simulink model "EENGquadcopter_control"  (R2018b)
settings: Solver=VariableStepAuto  StartTime=0.0  StopTime=10.0  RelTol=1e-3
values from neighbouring files (symbols this model uses):
  armLength = 0.1    [EENGquadcopter.m]
  dragFactor = 0.1    [EENGquadcopter.m]
  iX = 0.03    [EENGquadcopter.m]
  iY = 0.03    [EENGquadcopter.m]
  iZ = 0.03    [EENGquadcopter.m]
  mass = 0.25    [EENGquadcopter.m]
  om1 = 2.8    [EENGquadcopter.m]
  om2 = 3.2    [EENGquadcopter.m]
  om3 = 3.2    [EENGquadcopter.m]
  om4 = 2.8    [EENGquadcopter.m]
  phi0 = 0.0    (= 0)    [EENGquadcopter.m]    (also in EKFquadcopter-1.m = x_k0(4) + (e*(-1^count)); UKFquadcopter-1.m = xI_p(4,i))
  phiDot0 = 0.0    (= 0)    [EENGquadcopter.m]    (also in EKFquadcopter-1.m = x_k0(10) + (e*(-1^(count+1))); UKFquadcopter-1.m = xI_p(10,i))
  psi0 = 0.0    (= 0)    [EENGquadcopter.m]    (also in EKFquadcopter-1.m = x_k0(6) + (e*(-1^count)); UKFquadcopter-1.m = xI_p(6,i))
  psiDot0 = 0.0    (= 0)    [EENGquadcopter.m]    (also in EKFquadcopter-1.m = x_k0(12) + (e*(-1^(count+1))); UKFquadcopter-1.m = xI_p(12,i))
  theta0 = 0.0    (= 0)    [EENGquadcopter.m]    (also in EKFquadcopter-1.m = x_k0(5) + (e*(-1^(count+1))); UKFquadcopter-1.m = xI_p(5,i))
  thetaDot0 = 0.0    (= 0)    [EENGquadcopter.m]    (also in EKFquadcopter-1.m = x_k0(11) + (e*(-1^count)); UKFquadcopter-1.m = xI_p(11,i))
  thrustFactor = 0.1    [EENGquadcopter.m]
  Ts = 0.025    [EKFquadcopter-1.m]    (also in UKFquadcopter-1.m)
  x0 = 0.0    (= 0)    [EENGquadcopter.m]    (also in EKFquadcopter-1.m = x_k0(1) + e*(-1^count); UKFquadcopter-1.m = xI_p(1,i))
  xDot0 = 0.0    (= 0)    [EENGquadcopter.m]    (also in EKFquadcopter-1.m = x_k0(7) + (e*(-1^(count+1))); UKFquadcopter-1.m = xI_p(7,i))
  y0 = 0.0    (= 0)    [EENGquadcopter.m]    (also in EKFquadcopter-1.m = x_k0(2) + (e*(-1^(count+1))); UKFquadcopter-1.m = xI_p(2,i))
  yDot0 = 0.0    (= 0)    [EENGquadcopter.m]    (also in EKFquadcopter-1.m = x_k0(8) + (e*(-1^count)); UKFquadcopter-1.m = xI_p(8,i))
  z0 = 0.0    (= 0)    [EENGquadcopter.m]    (also in EKFquadcopter-1.m = x_k0(3) + (e*(-1^count)); UKFquadcopter-1.m = xI_p(3,i))
  zDot0 = 0.0    (= 0)    [EENGquadcopter.m]    (also in EKFquadcopter-1.m = x_k0(9) + (e*(-1^(count+1))); UKFquadcopter-1.m = xI_p(9,i))
libraries: simulink x1
settings Model: Creator=Ramprasad  LastModifiedBy=Ramprasad

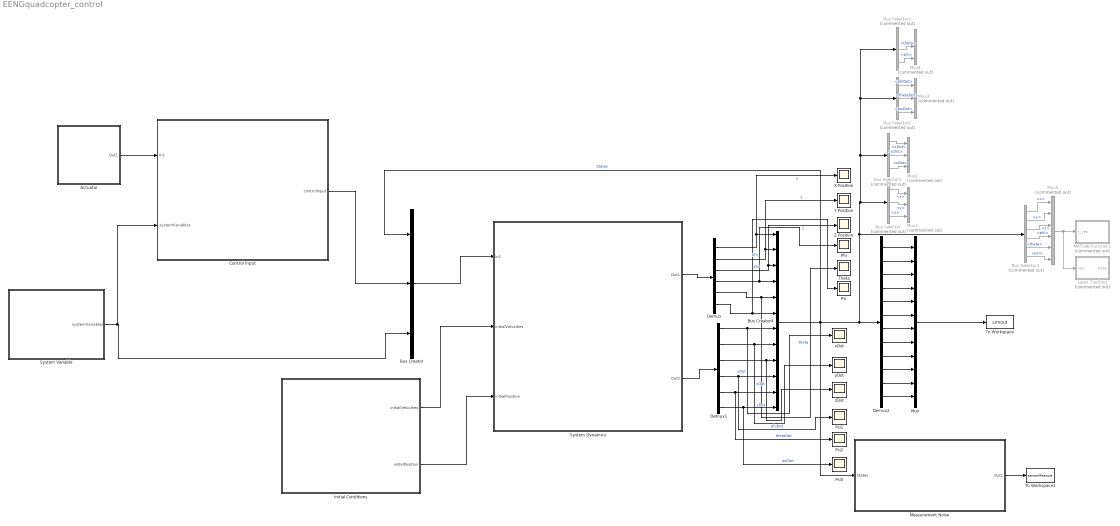
== system EENGquadcopter_control ==
  Actuator : Subsystem
  Bus Creator : BusCreator  Inputs=3
  Bus Creator4 : BusCreator  Inputs=12
  Bus Selector : BusSelector  Commented=on  OutputSignals=x,y,z
  Bus Selector1 : BusSelector  Commented=on  OutputSignals=xDot,yDot,zDot
  Bus Selector2 : BusSelector  Commented=on  OutputSignals=phiDot,thetaDot,psiDot
  Bus Selector3 : BusSelector  Commented=on  OutputSignals=phi,theta,psi
  Bus Selector4 : BusSelector  Commented=on  OutputSignals=x,y,z,phi,theta,psi
  Control Input : Subsystem
  Demux : Demux  Outputs=6
  Demux1 : Demux  Outputs=6
  Demux2 : Demux  Outputs=12
  Initial Conditions : Subsystem
  Laser Tracking : MATLAB Function  Commented=on  TreatAsAtomicUnit=on
  MATLAB Function1 : MATLAB Function  Commented=on  TreatAsAtomicUnit=on
  Measurement Noise : Subsystem
  Mux : Mux  Inputs=12
  Mux{1..4} (4 alike) : Mux  Commented=on  Inputs=3
  Mux5 : Mux  Commented=on  Inputs=6
  Phi : Scope
  Psi{,1..3} (4 alike) : Scope
  System Dynamics : Subsystem
  System Variable : Subsystem
  Theta : Scope
  To Workspace : ToWorkspace  VariableName=simout  SaveFormat=Timeseries  SampleTime=Ts
  To Workspace1 : ToWorkspace  VariableName=sensorMeasure  SaveFormat=Timeseries  SampleTime=-1
  X Position : Scope
  Y Position : Scope
  Z Position : Scope
  xDot : Scope
  yDot : Scope
  zDot : Scope
  wires:
  Demux/2 -> Bus Creator4/2, Y Position/1  "y"
  Bus Selector4/2 -> Mux5/2  "<y>"
  Demux2/8 -> Mux/8
  Bus Selector4/6 -> Mux5/6  "<psi>"
  Demux/6 -> Psi/1, Bus Creator4/6  "psi"
  Demux1/4 -> Psi1/1, Bus Creator4/10  "phiDot"
  Initial Conditions/2(initialPosition) -> System Dynamics/3(initialPosition)
  Measurement Noise/1(Out1) -> To Workspace1/1
  Bus Creator/1 -> System Dynamics/1(In1)
  Demux2/9 -> Mux/9
  Demux/3 -> Z Position/1, Bus Creator4/3  "z"
  Demux/4 -> Phi/1, Bus Creator4/4  "phi"
  System Dynamics/2(Out2) -> Demux1/1
  Demux2/12 -> Mux/12
  Demux2/7 -> Mux/7
  Demux2/6 -> Mux/6
  Demux1/5 -> Psi2/1, Bus Creator4/11  "thetaDot"
  Demux2/3 -> Mux/3
  Demux1/6 -> Psi3/1, Bus Creator4/12  "psiDot"
  Demux1/2 -> yDot/1, Bus Creator4/8  "yDot"
  Demux/1 -> Bus Creator4/1, X Position/1  "x"
  Demux/5 -> Theta/1, Bus Creator4/5  "theta"
  Demux2/10 -> Mux/10
  Bus Selector2/2 -> Mux3/2  "<thetaDot>"
  Demux1/1 -> xDot/1, Bus Creator4/7  "xDot"
  Bus Selector3/2 -> Mux4/2  "<theta>"
  Mux/1 -> To Workspace/1
  Bus Selector/3 -> Mux1/3  "<z>"
  Demux2/5 -> Mux/5
  Bus Selector2/3 -> Mux3/3  "<psiDot>"
  Demux2/2 -> Mux/2
  Bus Creator4/1 -> Bus Creator/1, Bus Selector3/1, Bus Selector2/1, Bus Selector1/1, Bus Selector/1, Bus Selector4/1, Demux2/1, Measurement Noise/1(States)  "States"
  Demux2/11 -> Mux/11
  Demux2/4 -> Mux/4
  System Variable/1(systemVariables) -> Control Input/2(systemVariables), Bus Creator/3
  Bus Selector/2 -> Mux1/2  "<y>"
  Demux1/3 -> zDot/1, Bus Creator4/9  "zDot"
  Bus Selector1/3 -> Mux2/3  "<zDot>"
  Bus Selector3/3 -> Mux4/3  "<psi>"
  Demux2/1 -> Mux/1
  Bus Selector1/1 -> Mux2/1  "<xDot>"
  System Dynamics/1(Out1) -> Demux/1
  Bus Selector1/2 -> Mux2/2  "<yDot>"
  Bus Selector4/1 -> Mux5/1  "<x>"
  Bus Selector/1 -> Mux1/1  "<x>"
  Mux5/1 -> Laser Tracking/1(xyz), MATLAB Function1/1(r_vec)
  Initial Conditions/1(initialVelocities) -> System Dynamics/2(initialVelocities)
  Bus Selector4/3 -> Mux5/3  "<z>"
  Bus Selector4/4 -> Mux5/4  "<phi>"
  Bus Selector4/5 -> Mux5/5  "<theta>"
  Bus Selector2/1 -> Mux3/1  "<phiDot>"
  Control Input/1(controlInput) -> Bus Creator/2
  Actuator/1(Out1) -> Control Input/1(In1)

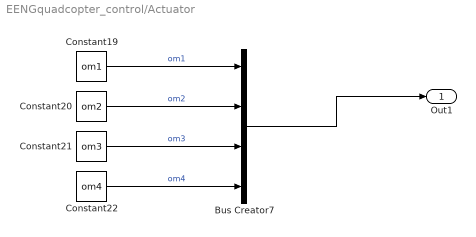
== system EENGquadcopter_control/Actuator ==
  Bus Creator7 : BusCreator  Inputs=4
  Constant19 : Constant  Value=om1
  Constant20 : Constant  Value=om2
  Constant21 : Constant  Value=om3
  Constant22 : Constant  Value=om4
  Out1 : Outport
  wires:
  Constant20/1 -> Bus Creator7/2  "om2"
  Bus Creator7/1 -> Out1/1
  Constant22/1 -> Bus Creator7/4  "om4"
  Constant21/1 -> Bus Creator7/3  "om3"
  Constant19/1 -> Bus Creator7/1  "om1"

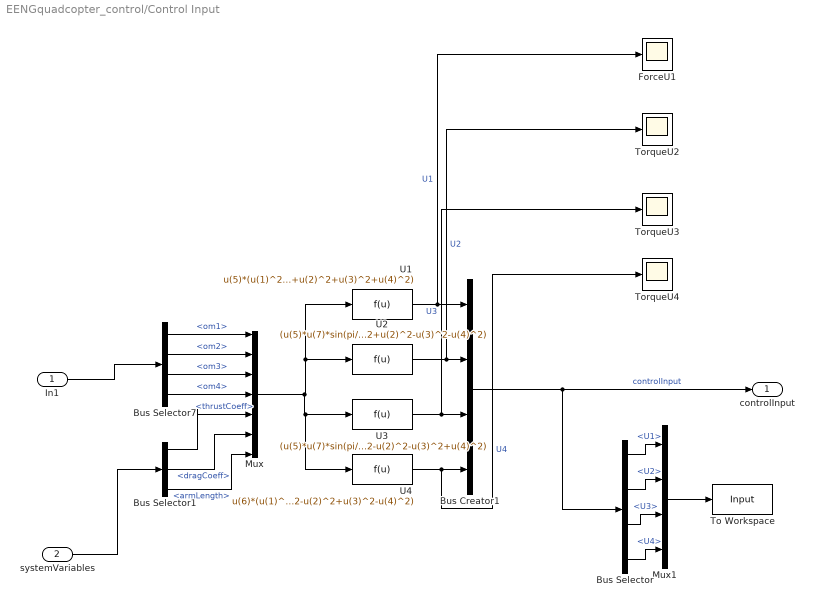
== system EENGquadcopter_control/Control Input ==
  In1 : Inport
  systemVariables : Inport  Port=2
  Bus Creator1 : BusCreator  Inputs=4
  Bus Selector : BusSelector  OutputSignals=U1,U2,U3,U4
  Bus Selector1 : BusSelector  OutputSignals=thrustCoeff,dragCoeff,armLength
  Bus Selector7 : BusSelector  OutputSignals=om1,om2,om3,om4
  ForceU1 : Scope
  Mux : Mux  Inputs=7
  Mux1 : Mux
  To Workspace : ToWorkspace  VariableName=Input  SaveFormat=Timeseries  SampleTime=-1
  TorqueU2 : Scope
  TorqueU3 : Scope
  TorqueU4 : Scope
  U1 : Fcn  Expr=u(5)*(u(1)^2+u(2)^2+u(3)^2+u(4)^2)
  U2 : Fcn  Expr=(u(5)*u(7)*sin(pi/4))*(u(1)^2+u(2)^2-u(3)^2-u(4)^2)
  U3 : Fcn  Expr=(u(5)*u(7)*sin(pi/4))*(u(1)^2-u(2)^2-u(3)^2+u(4)^2)
  U4 : Fcn  Expr=u(6)*(u(1)^2-u(2)^2+u(3)^2-u(4)^2)
  controlInput : Outport
  wires:
  systemVariables/1 -> Bus Selector1/1
  Bus Selector7/2 -> Mux/2  "<om2>"
  Bus Selector7/4 -> Mux/4  "<om4>"
  Bus Selector7/1 -> Mux/1  "<om1>"
  U2/1 -> TorqueU2/1, Bus Creator1/2  "U2"
  Bus Selector1/2 -> Mux/6  "<dragCoeff>"
  Bus Creator1/1 -> Bus Selector/1, controlInput/1  "controlInput"
  Bus Selector1/1 -> Mux/5  "<thrustCoeff>"
  U3/1 -> TorqueU3/1, Bus Creator1/3  "U3"
  Bus Selector1/3 -> Mux/7  "<armLength>"
  U4/1 -> TorqueU4/1, Bus Creator1/4  "U4"
  U1/1 -> ForceU1/1, Bus Creator1/1  "U1"
  Mux/1 -> U4/1, U3/1, U2/1, U1/1
  In1/1 -> Bus Selector7/1
  Bus Selector7/3 -> Mux/3  "<om3>"
  Bus Selector/1 -> Mux1/1  "<U1>"
  Bus Selector/2 -> Mux1/2  "<U2>"
  Bus Selector/3 -> Mux1/3  "<U3>"
  Bus Selector/4 -> Mux1/4  "<U4>"
  Mux1/1 -> To Workspace/1

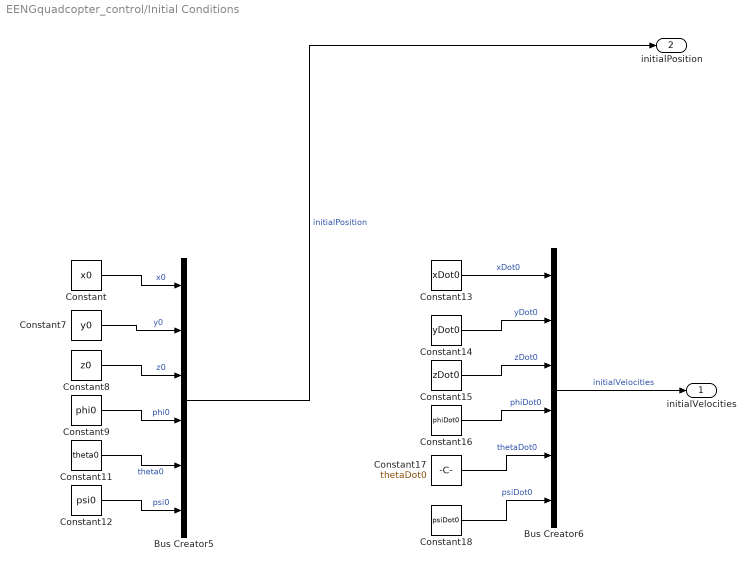
== system EENGquadcopter_control/Initial Conditions ==
  Bus Creator5 : BusCreator  Inputs=6
  Bus Creator6 : BusCreator  Inputs=6
  Constant : Constant  Value=x0
  Constant11 : Constant  Value=theta0
  Constant12 : Constant  Value=psi0
  Constant13 : Constant  Value=xDot0
  Constant14 : Constant  Value=yDot0
  Constant15 : Constant  Value=zDot0
  Constant16 : Constant  Value=phiDot0
  Constant17 : Constant  Value=thetaDot0
  Constant18 : Constant  Value=psiDot0
  Constant7 : Constant  Value=y0
  Constant8 : Constant  Value=z0
  Constant9 : Constant  Value=phi0
  initialVelocities : Outport
  initialPosition : Outport  Port=2
  wires:
  Constant9/1 -> Bus Creator5/4  "phi0"
  Constant14/1 -> Bus Creator6/2  "yDot0"
  Constant17/1 -> Bus Creator6/5  "thetaDot0"
  Constant18/1 -> Bus Creator6/6  "psiDot0"
  Constant13/1 -> Bus Creator6/1  "xDot0"
  Constant11/1 -> Bus Creator5/5  "theta0"
  Constant8/1 -> Bus Creator5/3  "z0"
  Constant16/1 -> Bus Creator6/4  "phiDot0"
  Constant12/1 -> Bus Creator5/6  "psi0"
  Constant15/1 -> Bus Creator6/3  "zDot0"
  Constant/1 -> Bus Creator5/1  "x0"
  Bus Creator6/1 -> initialVelocities/1  "initialVelocities"
  Constant7/1 -> Bus Creator5/2  "y0"
  Bus Creator5/1 -> initialPosition/1  "initialPosition"

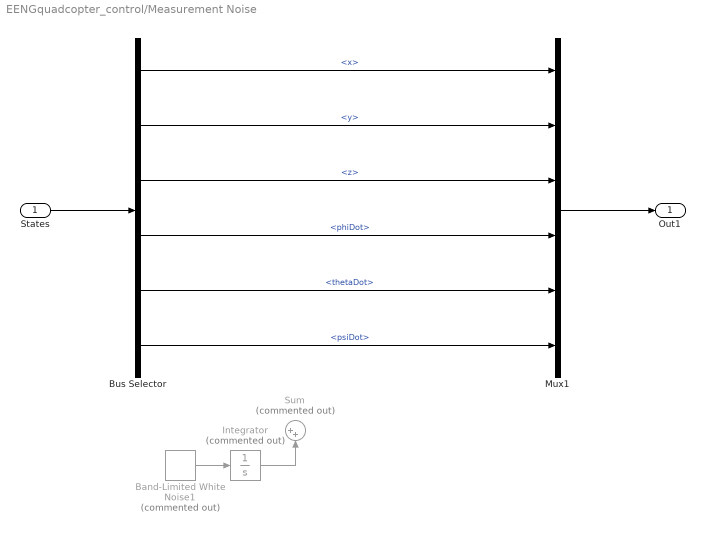
== system EENGquadcopter_control/Measurement Noise ==
  States : Inport
  Band-Limited White Noise1 : simulink/Sources/Band-Limited White Noise  Commented=on  Cov=[0.0]  Ts=Ts  seed=[23341]
  Bus Selector : BusSelector  OutputSignals=x,y,z,phiDot,thetaDot,psiDot
  Integrator : Integrator  Commented=on
  Mux1 : Mux  Inputs=6
  Sum : Sum  Commented=on  Inputs=|++
  Out1 : Outport
  wires:
  Integrator/1 -> Sum/2
  Bus Selector/3 -> Mux1/3  "<z>"
  Bus Selector/2 -> Mux1/2  "<y>"
  Mux1/1 -> Out1/1
  Band-Limited White Noise1/1 -> Integrator/1
  Bus Selector/4 -> Mux1/4  "<phiDot>"
  States/1 -> Bus Selector/1
  Bus Selector/6 -> Mux1/6  "<psiDot>"
  Bus Selector/5 -> Mux1/5  "<thetaDot>"
  Bus Selector/1 -> Mux1/1  "<x>"

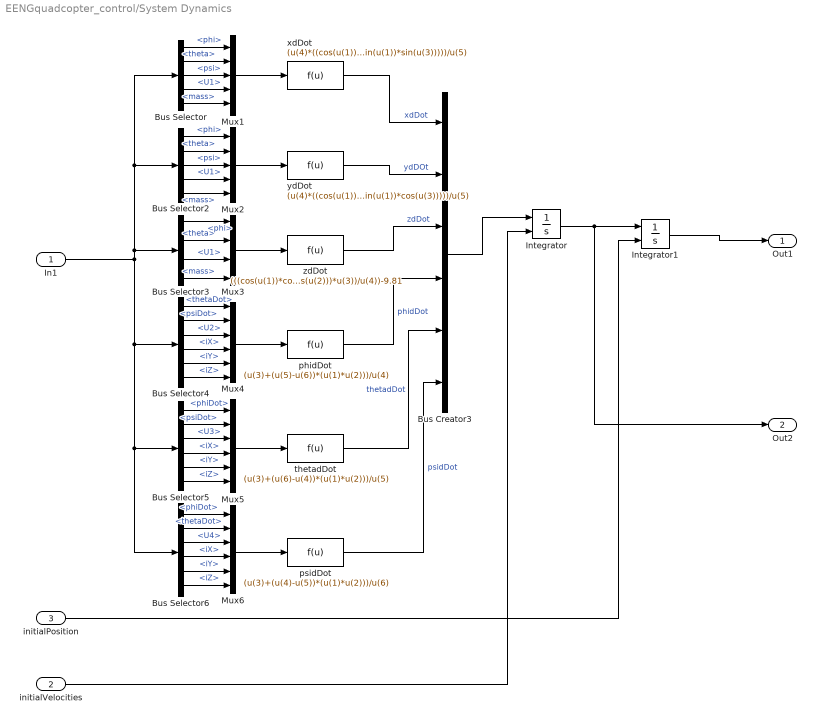
== system EENGquadcopter_control/System Dynamics ==
  In1 : Inport
  initialVelocities : Inport  Port=2
  initialPosition : Inport  Port=3
  Bus Creator3 : BusCreator  Inputs=6
  Bus Selector : BusSelector  OutputSignals=States.phi,States.theta,States.psi,controlInput.U1,systemVariables.mass
  Bus Selector2 : BusSelector  OutputSignals=States.phi,States.theta,States.psi,controlInput.U1,systemVariables.mass
  Bus Selector3 : BusSelector  OutputSignals=States.phi,States.theta,controlInput.U1,systemVariables.mass
  Bus Selector4 : BusSelector  OutputSignals=States.thetaDot,States.psiDot,controlInput.U2,systemVariables.iX,systemVariables.iY,systemVariables.iZ
  Bus Selector5 : BusSelector  OutputSignals=States.phiDot,States.psiDot,controlInput.U3,systemVariables.iX,systemVariables.iY,systemVariables.iZ
  Bus Selector6 : BusSelector  OutputSignals=States.phiDot,States.thetaDot,controlInput.U4,systemVariables.iX,systemVariables.iY,systemVariables.iZ
  Integrator : Integrator  InitialConditionSource=external
  Integrator1 : Integrator  InitialConditionSource=external
  Mux1 : Mux  Inputs=5
  Mux2 : Mux  Inputs=5
  Mux3 : Mux
  Mux4 : Mux  Inputs=6
  Mux5 : Mux  Inputs=6
  Mux6 : Mux  Inputs=6
  phidDot : Fcn  Expr=(u(3)+(u(5)-u(6))*(u(1)*u(2)))/u(4)
  psidDot : Fcn  Expr=(u(3)+(u(4)-u(5))*(u(1)*u(2)))/u(6)
  thetadDot : Fcn  Expr=(u(3)+(u(6)-u(4))*(u(1)*u(2)))/u(5)
  xdDot : Fcn  Expr=(u(4)*((cos(u(1))*sin(u(2))*cos(u(3)))+(sin(u(1))*sin(u(3)))))/u(5)
  ydDot : Fcn  Expr=(u(4)*((cos(u(1))*sin(u(2))*sin(u(3)))-(sin(u(1))*cos(u(3)))))/u(5)
  zdDot : Fcn  Expr=(((cos(u(1))*cos(u(2)))*u(3))/u(4))-9.81
  Out1 : Outport
  Out2 : Outport  Port=2
  wires:
  initialPosition/1 -> Integrator1/2
  xdDot/1 -> Bus Creator3/1  "xdDot"
  Bus Selector2/2 -> Mux2/2  "<theta>"
  Bus Selector4/5 -> Mux4/5  "<iY>"
  Bus Selector2/4 -> Mux2/4  "<U1>"
  Bus Selector4/3 -> Mux4/3  "<U2>"
  thetadDot/1 -> Bus Creator3/5  "thetadDot"
  Bus Selector5/2 -> Mux5/2  "<psiDot>"
  Bus Selector2/1 -> Mux2/1  "<phi>"
  Mux5/1 -> thetadDot/1
  Bus Selector6/4 -> Mux6/4  "<iX>"
  Bus Selector5/6 -> Mux5/6  "<iZ>"
  Bus Selector6/2 -> Mux6/2  "<thetaDot>"
  phidDot/1 -> Bus Creator3/4  "phidDot"
  Bus Selector2/3 -> Mux2/3  "<psi>"
  In1/1 -> Bus Selector4/1, Bus Selector5/1, Bus Selector6/1, Bus Selector3/1, Bus Selector2/1, Bus Selector/1
  Bus Selector5/3 -> Mux5/3  "<U3>"
  Bus Selector3/2 -> Mux3/2  "<theta>"
  Bus Selector3/1 -> Mux3/1  "<phi>"
  initialVelocities/1 -> Integrator/2
  Bus Selector/3 -> Mux1/3  "<psi>"
  Mux6/1 -> psidDot/1
  Bus Selector5/4 -> Mux5/4  "<iX>"
  Bus Selector/4 -> Mux1/4  "<U1>"
  Bus Selector/1 -> Mux1/1  "<phi>"
  Mux4/1 -> phidDot/1
  Bus Selector4/6 -> Mux4/6  "<iZ>"
  Bus Selector2/5 -> Mux2/5  "<mass>"
  Bus Creator3/1 -> Integrator/1
  Bus Selector6/6 -> Mux6/6  "<iZ>"
  Bus Selector3/3 -> Mux3/3  "<U1>"
  Mux2/1 -> ydDot/1
  Bus Selector6/3 -> Mux6/3  "<U4>"
  Bus Selector6/1 -> Mux6/1  "<phiDot>"
  zdDot/1 -> Bus Creator3/3  "zdDot"
  Bus Selector5/1 -> Mux5/1  "<phiDot>"
  Bus Selector4/2 -> Mux4/2  "<psiDot>"
  Bus Selector6/5 -> Mux6/5  "<iY>"
  Bus Selector4/4 -> Mux4/4  "<iX>"
  Bus Selector4/1 -> Mux4/1  "<thetaDot>"
  Mux3/1 -> zdDot/1
  Integrator/1 -> Integrator1/1, Out2/1
  psidDot/1 -> Bus Creator3/6  "psidDot"
  Integrator1/1 -> Out1/1
  Bus Selector/5 -> Mux1/5  "<mass>"
  ydDot/1 -> Bus Creator3/2  "ydDOt"
  Bus Selector5/5 -> Mux5/5  "<iY>"
  Bus Selector/2 -> Mux1/2  "<theta>"
  Bus Selector3/4 -> Mux3/4  "<mass>"
  Mux1/1 -> xdDot/1

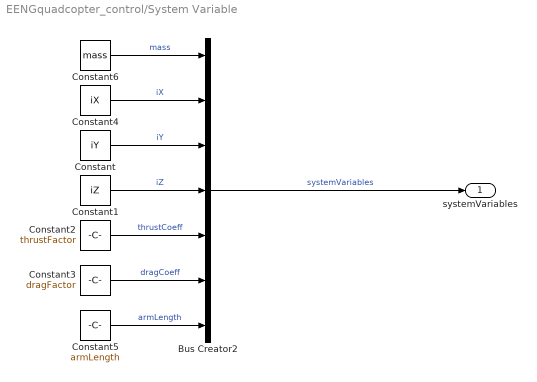
== system EENGquadcopter_control/System Variable ==
  Bus Creator2 : BusCreator  Inputs=7
  Constant : Constant  Value=iY
  Constant1 : Constant  Value=iZ
  Constant2 : Constant  Value=thrustFactor
  Constant3 : Constant  Value=dragFactor
  Constant4 : Constant  Value=iX
  Constant5 : Constant  Value=armLength
  Constant6 : Constant  Value=mass
  systemVariables : Outport
  wires:
  Constant6/1 -> Bus Creator2/1  "mass"
  Constant2/1 -> Bus Creator2/5  "thrustCoeff"
  Constant/1 -> Bus Creator2/3  "iY"
  Constant1/1 -> Bus Creator2/4  "iZ"
  Constant3/1 -> Bus Creator2/6  "dragCoeff"
  Constant4/1 -> Bus Creator2/2  "iX"
  Constant5/1 -> Bus Creator2/7  "armLength"
  Bus Creator2/1 -> systemVariables/1  "systemVariables"

== matlab function EENGquadcopter_control/MATLAB Function1 ==
  settings: updateMethod=DISCRETE
  data: r_vec input
function drawDrone(r_vec)
%#codegen
coder.extrinsic('evalin');
coder.extrinsic('load');
coder.extrinsic('animatedline');
% persistent figNum axisHandel Sim_Exact points3D;

% if isempty(Sim_Exact)
%     Sim_Exact = evalin('base','Sim_Exact');
%     a.points3D = zeros(21,3,'double');
%     a = load('points3D.mat');
%     points3D = zeros(21,3,'double');
%     points3D = a.points3D;
% end

x = r_vec(1);
y = r_vec(2);
z = r_vec(3);
phi = r_vec(4);
theta = r_vec(5);
psi = r_vec(6);

T06 = [cos(psi)*cos(theta) (cos(psi)*sin(theta)*sin(phi))-(sin(psi)*cos(phi)) (cos(phi)*sin(theta)*cos(psi))+(sin(phi)*sin(psi)) x;...
       sin(psi)*cos(theta) (sin(phi)*sin(theta)*sin(psi))+(cos(phi)*cos(psi)) (sin(psi)*sin(theta)*cos(phi))-(cos(psi)*sin(phi)) y;...
       -sin(theta) (cos(theta)*sin(phi)) (cos(theta)*cos(phi)) z;...
       0 0 0 1];

R06 = T06(1:3,1:3);

% P1 =[ 0
%     0
%     0.29];
% P2 = [ 0.27*cos(x)*cos(y);
%     0.27*cos(y)*sin(x);
%     0.29 - 0.27*sin(y)];
% P3 = [ 0.27*cos(x)*cos(y) - 0.07*cos(x)*sin(y)*sin(z) + 0.07*cos(x)*cos(y)*cos(z);
%     0.27*cos(y)*sin(x) - 0.07*sin(x)*sin(y)*sin(z) + 0.07*cos(y)*cos(z)*sin(x);
%     0.29 - 0.07*cos(y)*sin(z) - 0.07*cos(z)*sin(y) - 0.27*sin(y)];
% 
% P4 = [ 0.27*cos(x)*cos(y) - 0.07*cos(x)*sin(y)*sin(z) + 0.07*cos(x)*cos(y)*cos(z) - 0.302*cos(x)*cos(y)*sin(z) - 0.302*cos(x)*cos(z)*sin(y);
%     0.27*cos(y)*sin(x) - 0.302*cos(y)*sin(x)*sin(z) - 0.302*cos(z)*sin(x)*sin(y) - 0.07*sin(x)*sin(y)*sin(z) + 0.07*cos(y)*cos(z)*sin(x);
%     0.302*sin(y)*sin(z) - 0.302*cos(y)*cos(z) - 0.07*cos(y)*sin(z) - 0.07*cos(z)*sin(y) - 0.27*sin(y) + 0.29];
% P5 = [ 0.27*cos(x)*cos(y) - 0.07*cos(x)*sin(y)*sin(z) + 0.07*cos(x)*cos(y)*cos(z) - 0.302*cos(x)*cos(y)*sin(z) - 0.302*cos(x)*cos(z)*sin(y)
%     0.27*cos(y)*sin(x) - 0.302*cos(y)*sin(x)*sin(z) - 0.302*cos(z)*sin(x)*sin(y) - 0.07*sin(x)*sin(y)*sin(z) + 0.07*cos(y)*cos(z)*sin(x)
%     0.302*sin(y)*sin(z) - 0.302*cos(y)*cos(z) - 0.07*cos(y)*sin(z) - 0.07*cos(z)*sin(y) - 0.27*sin(y) + 0.29];
% 
% P6 =[ 0.27*cos(x)*cos(y) - 0.07*cos(x)*sin(y)*sin(z) - 0.072*sin(x)*sin(phi)*sin(theta) + 0.07*cos(x)*cos(y)*cos(z) - 0.302*cos(x)*cos(y)*sin(z) - 0.302*cos(x)*cos(z)*sin(y) - 0.072*cos(x)*cos(y)*cos(theta)*sin(z) - 0.072*cos(x)*cos(z)*cos(theta)*sin(y) - 0.072*cos(x)*cos(y)*cos(z)*cos(phi)*sin(theta) + 0.072*cos(x)*cos(phi)*sin(y)*sin(z)*sin(theta);
%     0.27*cos(y)*sin(x) - 0.302*cos(y)*sin(x)*sin(z) - 0.302*cos(z)*sin(x)*sin(y) + 0.072*cos(x)*sin(phi)*sin(theta) - 0.07*sin(x)*sin(y)*sin(z) + 0.07*cos(y)*cos(z)*sin(x) - 0.072*cos(y)*cos(theta)*sin(x)*sin(z) - 0.072*cos(z)*cos(theta)*sin(x)*sin(y) - 0.072*cos(y)*cos(z)*cos(phi)*sin(x)*sin(theta) + 0.072*cos(phi)*sin(x)*sin(y)*sin(z)*sin(theta);
%     0.302*sin(y)*sin(z) - 0.302*cos(y)*cos(z) - 0.07*cos(y)*sin(z) - 0.07*cos(z)*sin(y) - 0.27*sin(y) + 0.072*cos(theta)*sin(y)*sin(z) - 0.072*cos(y)*cos(z)*cos(theta) + 0.072*cos(y)*cos(phi)*sin(z)*sin(theta) + 0.072*cos(z)*cos(phi)*sin(y)*sin(theta) + 0.29];

Q1 = [(0.1/sqrt(2));(0.1/sqrt(2));0];
Q2 = [-(0.1/sqrt(2));(0.1/sqrt(2));0];
Q3 = [(0.1/sqrt(2));-(0.1/sqrt(2));0];
Q4 = [-(0.1/sqrt(2));-(0.1/sqrt(2));0];

R1 = R06*Q1;
R2 = R06*Q2;
R3 = R06*Q3;
R4 = R06*Q4;

P1 = [x+R1(1);y+R1(2);z+R1(3)];
P2 = [x+R2(1);y+R2(2);z+R2(3)];
P3 = [x+R3(1);y+R3(2);z+R3(3)];
P4 = [x+R4(1);y+R4(2);z+R4(3)];

% if isempty(figNum)
%     figNum = figure(1);
%     hold on;
%     plot3([0;P1(1);P2(1);P3(1);P4(1);P5(1);P6(1)],...
%         [0;P1(2);P2(2);P3(2);P4(2);P5(2);P6(2)],...
%         [0;P1(3);P2(3);P3(3);P4(3);P5(3);P6(3)],'k','linewidth',2);
%     axisHandel = gca;
%     plot3([P6(1);P6(1)+T06(1,1)*.1],...
%         [P6(2);P6(2)+T06(2,1)*.1],...
%         [P6(3);P6(3)+T06(3,1)*.1],'r','Parent',axisHandel);
%     plot3([P6(1);P6(1)+T06(1,2)*.1],...
%         [P6(2);P6(2)+T06(2,2)*.1],...
%         [P6(3);P6(3)+T06(3,2)*.1],'g','Parent',axisHandel);
%     plot3([P6(1);P6(1)+T06(1,3)*.1],...
%         [P6(2);P6(2)+T06(2,3)*.1],...
%         [P6(3);P6(3)+T06(3,3)*.1],'b','Parent',axisHandel);
%     plot3(points3D(:,1),points3D(:,2),points3D(:,3),'m','Parent',axisHandel);
%     hold off;
%     axis([-.75 .75 -.75 .75 -.4 .75]);
%     axisHandel = gca;
% else
figure(1)
plot3([x;P1(1)],[y;P1(2)],[z;P1(3)],'k','linewidth',2,'Parent',gca);
hold on;
plot3([x;P2(1)],[y;P2(2)],[z;P2(3)],'k','linewidth',2,'Parent',gca);
hold on;
plot3([x;P3(1)],[y;P3(2)],[z;P3(3)],'k','linewidth',2,'Parent',gca);
hold on;
plot3([x;P4(1)],[y;P4(2)],[z;P4(3)],'k','linewidth',2,'Parent',gca);
hold on;
plot3([x;x+T06(1,1)*.1],[y;y+T06(2,1)*.1],[z;z+T06(3,1)*.1],'r','Parent',gca);
plot3([x;x+T06(1,2)*.1],[y;y+T06(2,2)*.1],[z;z+T06(3,2)*.1],'g','Parent',gca);
plot3([x;x+T06(1,3)*.1],[y;y+T06(2,3)*.1],[z;z+T06(3,3)*.1],'b','Parent',gca);
% plot3([P6(1);P6(1)+T06(1,2)*.1],...
%     [P6(2);P6(2)+T06(2,2)*.1],...
%     [P6(3);P6(3)+T06(3,2)*.1],'g','Parent',gca);
% plot3([P6(1);P6(1)+T06(1,3)*.1],...
%     [P6(2);P6(2)+T06(2,3)*.1],...
%     [P6(3);P6(3)+T06(3,3)*.1],'b','Parent',gca);
% plot3(x,y,z,'m','Parent',gca);
hold off;
axis([-0.1 1.1 -0.1 1.1 0.0 1.1]);
end

== matlab function EENGquadcopter_control/Laser Tracking ==
  data: xyz input; pose output
function pose = laserTracker(xyz)
%#codegen
coder.extrinsic('evalin');
% persistent Sim_Exact;
% 
% if isempty(Sim_Exact)
%     Sim_Exact = evalin('base','Sim_Exact');
% end


x = xyz(1,1);
y = xyz(2,1);
z = xyz(3,1);
    
% pose = [ sin(th6)*(cos(th4)*sin(th1) + sin(th4)*(cos(th1)*sin(th2)*sin(th3) - cos(th1)*cos(th2)*cos(th3))) + cos(th6)*(cos(th5)*(sin(th1)*sin(th4) - cos(th4)*(cos(th1)*sin(th2)*sin(th3) - cos(th1)*cos(th2)*cos(th3))) - sin(th5)*(cos(th1)*cos(th2)*sin(th3) + cos(th1)*cos(th3)*sin(th2))), cos(th6)*(cos(th4)*sin(th1) + sin(th4)*(cos(th1)*sin(th2)*sin(th3) - cos(th1)*cos(th2)*cos(th3))) - sin(th6)*(cos(th5)*(sin(th1)*sin(th4) - cos(th4)*(cos(th1)*sin(th2)*sin(th3) - cos(th1)*cos(th2)*cos(th3))) - sin(th5)*(cos(th1)*cos(th2)*sin(th3) + cos(th1)*cos(th3)*sin(th2))), - sin(th5)*(sin(th1)*sin(th4) - cos(th4)*(cos(th1)*sin(th2)*sin(th3) - cos(th1)*cos(th2)*cos(th3))) - cos(th5)*(cos(th1)*cos(th2)*sin(th3) + cos(th1)*cos(th3)*sin(th2)), (151838081588107*cos(th1)*cos(th2))/562949953421312 - (123928564092639*sin(th1))/72057594037927936 - (7184037743251309*cos(th1))/36893488147419103232 - (7330531551818703*cos(th4)*sin(th1))/36893488147419103232 - (5489399374888815*sin(th1)*sin(th4))/9223372036854775808 + (970893499285375*cos(th5)*(sin(th1)*sin(th4) - cos(th4)*(cos(th1)*sin(th2)*sin(th3) - cos(th1)*cos(th2)*cos(th3))))/9223372036854775808 - (5192391675427195*sin(th5)*(sin(th1)*sin(th4) - cos(th4)*(cos(th1)*sin(th2)*sin(th3) - cos(th1)*cos(th2)*cos(th3))))/72057594037927936 + (1663072680156839*sin(th6)*(cos(th4)*sin(th1) + sin(th4)*(cos(th1)*sin(th2)*sin(th3) - cos(th1)*cos(th2)*cos(th3))))/2305843009213693952 + (1663072680156839*cos(th6)*(cos(th5)*(sin(th1)*sin(th4) - cos(th4)*(cos(th1)*sin(th2)*sin(th3) - cos(th1)*cos(th2)*cos(th3))) - sin(th5)*(cos(th1)*cos(th2)*sin(th3) + cos(th1)*cos(th3)*sin(th2))))/2305843009213693952 + (5489399374888815*cos(th4)*(cos(th1)*sin(th2)*sin(th3) - cos(th1)*cos(th2)*cos(th3)))/9223372036854775808 - (5192391675427195*cos(th5)*(cos(th1)*cos(th2)*sin(th3) + cos(th1)*cos(th3)*sin(th2)))/72057594037927936 - (7330531551818703*sin(th4)*(cos(th1)*sin(th2)*sin(th3) - cos(th1)*cos(th2)*cos(th3)))/36893488147419103232 - (970893499285375*sin(th5)*(cos(th1)*cos(th2)*sin(th3) + cos(th1)*cos(th3)*sin(th2)))/9223372036854775808 - (1259578569946919*cos(th1)*sin(th2)*sin(th3))/18014398509481984 + (1259578569946919*cos(th1)*cos(th2)*cos(th3))/18014398509481984 - (5430591396830085*cos(th1)*cos(th2)*sin(th3))/18014398509481984 - (5430591396830085*cos(th1)*cos(th3)*sin(th2))/18014398509481984;
%     - sin(th6)*(cos(th1)*cos(th4) - sin(th4)*(sin(th1)*sin(th2)*sin(th3) - cos(th2)*cos(th3)*sin(th1))) - cos(th6)*(cos(th5)*(cos(th1)*sin(th4) + cos(th4)*(sin(th1)*sin(th2)*sin(th3) - cos(th2)*cos(th3)*sin(th1))) + sin(th5)*(cos(th2)*sin(th1)*sin(th3) + cos(th3)*sin(th1)*sin(th2))), sin(th6)*(cos(th5)*(cos(th1)*sin(th4) + cos(th4)*(sin(th1)*sin(th2)*sin(th3) - cos(th2)*cos(th3)*sin(th1))) + sin(th5)*(cos(th2)*sin(th1)*sin(th3) + cos(th3)*sin(th1)*sin(th2))) - cos(th6)*(cos(th1)*cos(th4) - sin(th4)*(sin(th1)*sin(th2)*sin(th3) - cos(th2)*cos(th3)*sin(th1))), sin(th5)*(cos(th1)*sin(th4) + cos(th4)*(sin(th1)*sin(th2)*sin(th3) - cos(th2)*cos(th3)*sin(th1))) - cos(th5)*(cos(th2)*sin(th1)*sin(th3) + cos(th3)*sin(th1)*sin(th2)), (123928564092639*cos(th1))/72057594037927936 - (7184037743251309*sin(th1))/36893488147419103232 + (7330531551818703*cos(th1)*cos(th4))/36893488147419103232 + (151838081588107*cos(th2)*sin(th1))/562949953421312 + (5489399374888815*cos(th1)*sin(th4))/9223372036854775808 - (970893499285375*cos(th5)*(cos(th1)*sin(th4) + cos(th4)*(sin(th1)*sin(th2)*sin(th3) - cos(th2)*cos(th3)*sin(th1))))/9223372036854775808 + (5192391675427195*sin(th5)*(cos(th1)*sin(th4) + cos(th4)*(sin(th1)*sin(th2)*sin(th3) - cos(th2)*cos(th3)*sin(th1))))/72057594037927936 - (1663072680156839*sin(th6)*(cos(th1)*cos(th4) - sin(th4)*(sin(th1)*sin(th2)*sin(th3) - cos(th2)*cos(th3)*sin(th1))))/2305843009213693952 + (5489399374888815*cos(th4)*(sin(th1)*sin(th2)*sin(th3) - cos(th2)*cos(th3)*sin(th1)))/9223372036854775808 - (5192391675427195*cos(th5)*(cos(th2)*sin(th1)*sin(th3) + cos(th3)*sin(th1)*sin(th2)))/72057594037927936 - (1663072680156839*cos(th6)*(cos(th5)*(cos(th1)*sin(th4) + cos(th4)*(sin(th1)*sin(th2)*sin(th3) - cos(th2)*cos(th3)*sin(th1))) + sin(th5)*(cos(th2)*sin(th1)*sin(th3) + cos(th3)*sin(th1)*sin(th2))))/2305843009213693952 - (7330531551818703*sin(th4)*(sin(th1)*sin(th2)*sin(th3) - cos(th2)*cos(th3)*sin(th1)))/36893488147419103232 - (970893499285375*sin(th5)*(cos(th2)*sin(th1)*sin(th3) + cos(th3)*sin(th1)*sin(th2)))/9223372036854775808 - (5430591396830085*cos(th2)*sin(th1)*sin(th3))/18014398509481984 - (5430591396830085*cos(th3)*sin(th1)*sin(th2))/18014398509481984 - (1259578569946919*sin(th1)*sin(th2)*sin(th3))/18014398509481984 + (1259578569946919*cos(th2)*cos(th3)*sin(th1))/18014398509481984;
%     sin(th4)*sin(th6)*(cos(th2)*sin(th3) + cos(th3)*sin(th2)) - cos(th6)*(sin(th5)*(cos(th2)*cos(th3) - sin(th2)*sin(th3)) + cos(th4)*cos(th5)*(cos(th2)*sin(th3) + cos(th3)*sin(th2))), sin(th6)*(sin(th5)*(cos(th2)*cos(th3) - sin(th2)*sin(th3)) + cos(th4)*cos(th5)*(cos(th2)*sin(th3) + cos(th3)*sin(th2))) + cos(th6)*sin(th4)*(cos(th2)*sin(th3) + cos(th3)*sin(th2)), cos(th4)*sin(th5)*(cos(th2)*sin(th3) + cos(th3)*sin(th2)) - cos(th5)*(cos(th2)*cos(th3) - sin(th2)*sin(th3)), (5430591396830085*sin(th2)*sin(th3))/18014398509481984 - (5430591396830085*cos(th2)*cos(th3))/18014398509481984 - (1259578569946919*cos(th2)*sin(th3))/18014398509481984 - (1259578569946919*cos(th3)*sin(th2))/18014398509481984 - (1663072680156839*cos(th6)*(sin(th5)*(cos(th2)*cos(th3) - sin(th2)*sin(th3)) + cos(th4)*cos(th5)*(cos(th2)*sin(th3) + cos(th3)*sin(th2))))/2305843009213693952 - (151838081588107*sin(th2))/562949953421312 + (5489399374888815*cos(th4)*(cos(th2)*sin(th3) + cos(th3)*sin(th2)))/9223372036854775808 - (5192391675427195*cos(th5)*(cos(th2)*cos(th3) - sin(th2)*sin(th3)))/72057594037927936 - (7330531551818703*sin(th4)*(cos(th2)*sin(th3) + cos(th3)*sin(th2)))/36893488147419103232 - (970893499285375*sin(th5)*(cos(th2)*cos(th3) - sin(th2)*sin(th3)))/9223372036854775808 - (970893499285375*cos(th4)*cos(th5)*(cos(th2)*sin(th3) + cos(th3)*sin(th2)))/9223372036854775808 + (5192391675427195*cos(th4)*sin(th5)*(cos(th2)*sin(th3) + cos(th3)*sin(th2)))/72057594037927936 + (1663072680156839*sin(th4)*sin(th6)*(cos(th2)*sin(th3) + cos(th3)*sin(th2)))/2305843009213693952 + 325695105792877/1125899906842624;
%     0, 0, 0, 1];

pose = [x;y;z];
end
